simulink model "Robot_Protected_Model"  (Simulink 8.0)
settings: Solver=ode45  StartTime=0.0  StopTime=simtime  MaxStep=0.01  RelTol=1e-3
values from neighbouring files (symbols this model uses):
  de = 30*pi/180    (= 0.523598775598)    [Robot_Feedback_Master.m]
  de0 = 0    [Robot_Feedback_Master.m]
  F = [mu1, 0; 0, mu2]    [Robot_Feedback_Master.m]
  g = 9.81    [Robot_Feedback_Master.m]
  Gamma0 = 1*diag([1, 1, 1, 1, 1, 1, 1, 1, 1], 0)    [Robot_Feedback_Master.m]
  Gamma1 = 0.0*diag([1, 1, 1, 1, 1, 1, 1, 1, 1], 0)    [Robot_Feedback_Master.m]
  I1 = 0.12    [Robot_Feedback_Master.m]
  Ie = 0.25    [Robot_Feedback_Master.m]
  Ie0 = 0.12    [Robot_Feedback_Master.m]
  initial_pos = 1*[-3; -3]    [Robot_Feedback_Master.m]
  initial_theta = 0*theta'    [Robot_Feedback_Master.m]
  initial_vel = 1*[-6; 6]    [Robot_Feedback_Master.m]
  KD = 100 * eye(2, 2)    [Robot_Feedback_Master.m]
  L1 = 1    [Robot_Feedback_Master.m]
  lambda = 0    [Robot_Feedback_Master.m]
  Lambda = 10 * eye(2, 2)    [Robot_Feedback_Master.m]
  Lc1 = 0.5    [Robot_Feedback_Master.m]
  Lce = 0.6    [Robot_Feedback_Master.m]
  Lce0 = 0.5    [Robot_Feedback_Master.m]
  M1 = 1    [Robot_Feedback_Master.m]
  Me = 5    [Robot_Feedback_Master.m]
  Me0 = 1    [Robot_Feedback_Master.m]
  mu1 = 0*0.1    (= 0)    [Robot_Feedback_Master.m]
  mu10 = 0*0.2    (= 0)    [Robot_Feedback_Master.m]
  mu2 = 0*0.1    (= 0)    [Robot_Feedback_Master.m]
  mu20 = 0*0.2    (= 0)    [Robot_Feedback_Master.m]
  tau1lim = 500    [Robot_Feedback_Master.m]
  tau2lim = 250    [Robot_Feedback_Master.m]
  thetaeps = 10    [Robot_Feedback_Master.m]
  thetamax = 40    [Robot_Feedback_Master.m]
settings Model: Creator=Travis  LastModifiedBy=Dan
settings DataIOCC: SignalLoggingSaveFormat=ModelDataLogs
settings DebuggingCC: FcnCallInpInsideContextMsg=UseLocalSettings
settings GRTTargetCC: CombineOutputUpdateFcns=off  GRTInterface=on

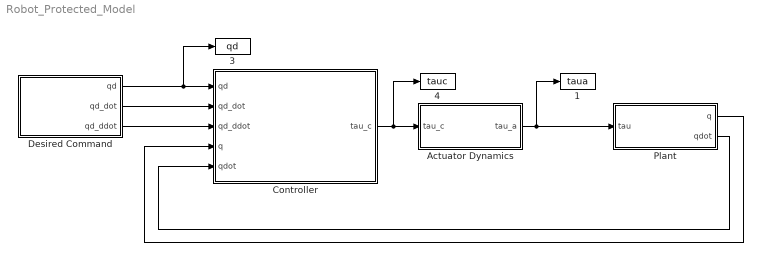
== system Robot_Protected_Model ==
  1 : ToWorkspace  VariableName=taua  SampleTime=-1  SaveFormat=Structure With Time
  3 : ToWorkspace  VariableName=qd  SampleTime=-1  SaveFormat=Structure With Time
  4 : ToWorkspace  VariableName=tauc  SampleTime=-1  SaveFormat=Structure With Time
  Actuator Dynamics : Subsystem
  Controller : Subsystem
  Desired Command : Subsystem
  Plant : Subsystem
  wires:
  Plant/2(qdot) -> Controller/5(qdot)
  Plant/1(q) -> Controller/4(q)
  Controller/1(tau_c) -> 4/1, Actuator Dynamics/1(tau_c)
  Desired Command/1(qd) -> 3/1, Controller/1(qd)
  Actuator Dynamics/1(tau_a) -> Plant/1(tau), 1/1
  Desired Command/2(qd_dot) -> Controller/2(qd_dot)
  Desired Command/3(qd_ddot) -> Controller/3(qd_ddot)

== system Robot_Protected_Model/Actuator Dynamics ==
  tau_c : Inport
  Demux : Demux  Outputs=2
  Mux : Mux  Inputs=2
  Saturation : Saturate  UpperLimit=tau1lim  LowerLimit=-tau1lim  ZeroCross=off
  Saturation1 : Saturate  UpperLimit=tau2lim  LowerLimit=-tau2lim  ZeroCross=off
  tau_a : Outport
  wires:
  Demux/1 -> Saturation/1
  Saturation/1 -> Mux/1
  Demux/2 -> Saturation1/1
  Saturation1/1 -> Mux/2
  Mux/1 -> tau_a/1
  tau_c/1 -> Demux/1

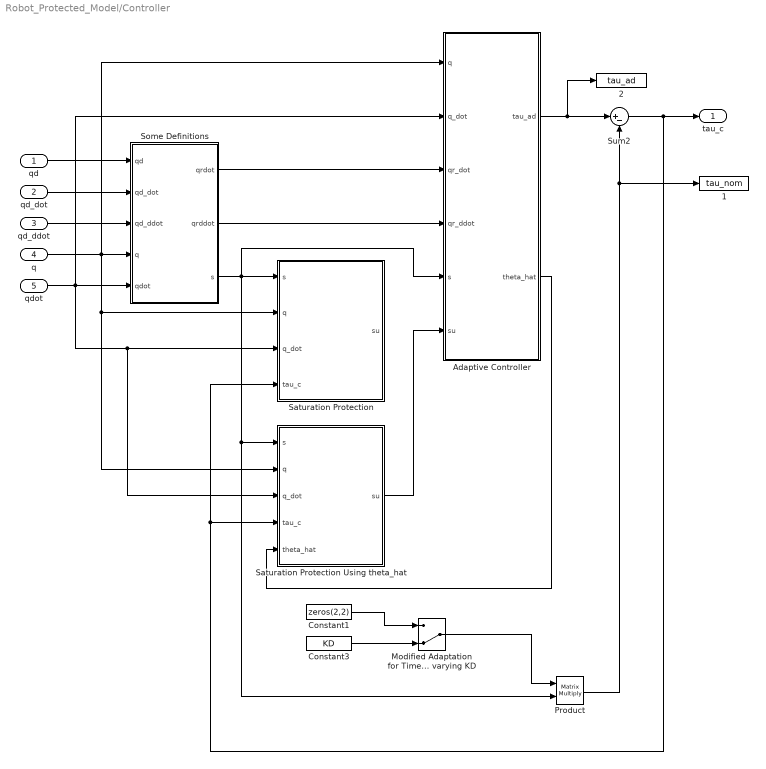
== system Robot_Protected_Model/Controller ==
  qd : Inport
  qd_dot : Inport  Port=2
  qd_ddot : Inport  Port=3
  q : Inport  Port=4
  qdot : Inport  Port=5
  1 : ToWorkspace  VariableName=tau_nom  SampleTime=-1  SaveFormat=Structure With Time
  2 : ToWorkspace  VariableName=tau_ad  SampleTime=-1  SaveFormat=Structure With Time
  Adaptive Controller : Subsystem
  Constant1 : Constant  Value=zeros(2,2)
  Constant3 : Constant  Value=KD
  Modified Adaptation for Time Varying KD (SWITCH 2 of 2) up is time varying KD : ManualSwitch  CurrentSetting=0
  Product : Product  Multiplication=Matrix(*)  RndMeth=Zero
  Saturation Protection : Subsystem
  Saturation Protection Using theta_hat : Subsystem
  Some Definitions : Subsystem
  Sum2 : Sum  Inputs=|+-
  tau_c : Outport
  wires:
  Adaptive Controller/1(tau_ad) -> 2/1, Sum2/1
  Product/1 -> 1/1, Sum2/2
  Sum2/1 -> tau_c/1, Saturation Protection/4(tau_c), Saturation Protection Using theta_hat/4(tau_c)
  q/1 -> Saturation Protection Using theta_hat/2(q), Saturation Protection/2(q), Some Definitions/4(q), Adaptive Controller/1(q)
  qdot/1 -> Adaptive Controller/2(q_dot), Saturation Protection Using theta_hat/3(q_dot), Saturation Protection/3(q_dot), Some Definitions/5(qdot)
  Some Definitions/1(qrdot) -> Adaptive Controller/3(qr_dot)
  Some Definitions/2(qrddot) -> Adaptive Controller/4(qr_ddot)
  qd_ddot/1 -> Some Definitions/3(qd_ddot)
  qd_dot/1 -> Some Definitions/2(qd_dot)
  qd/1 -> Some Definitions/1(qd)
  Some Definitions/3(s) -> Saturation Protection Using theta_hat/1(s), Product/2, Adaptive Controller/5(s), Saturation Protection/1(s)
  Constant3/1 -> Modified Adaptation for Time Varying KD (SWITCH 2 of 2) up is time varying KD/2
  Constant1/1 -> Modified Adaptation for Time Varying KD (SWITCH 2 of 2) up is time varying KD/1
  Modified Adaptation for Time Varying KD (SWITCH 2 of 2) up is time varying KD/1 -> Product/1
  Adaptive Controller/2(theta_hat) -> Saturation Protection Using theta_hat/5(theta_hat)
  Saturation Protection Using theta_hat/1(su) -> Adaptive Controller/6(su)

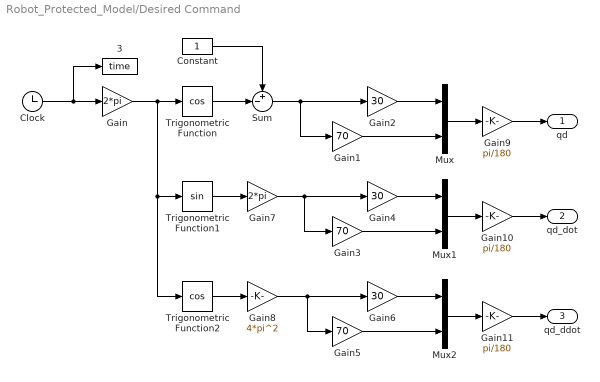
== system Robot_Protected_Model/Desired Command ==
  3 : ToWorkspace  VariableName=time  SampleTime=-1
  Clock : Clock
  Constant : Constant
  Gain : Gain  Gain=2*pi
  Gain1 : Gain  Gain=70
  Gain10 : Gain  Gain=pi/180
  Gain11 : Gain  Gain=pi/180
  Gain2 : Gain  Gain=30
  Gain3 : Gain  Gain=70
  Gain4 : Gain  Gain=30
  Gain5 : Gain  Gain=70
  Gain6 : Gain  Gain=30
  Gain7 : Gain  Gain=2*pi
  Gain8 : Gain  Gain=4*pi^2
  Gain9 : Gain  Gain=pi/180
  Mux : Mux  Inputs=2
  Mux1 : Mux  Inputs=2
  Mux2 : Mux  Inputs=2
  Sum : Sum  Inputs=+-|
  Trigonometric Function : Trigonometry  Operator=cos
  Trigonometric Function1 : Trigonometry
  Trigonometric Function2 : Trigonometry  Operator=cos
  qd : Outport
  qd_dot : Outport  Port=2
  qd_ddot : Outport  Port=3
  wires:
  Clock/1 -> Gain/1, 3/1
  Gain/1 -> Trigonometric Function/1, Trigonometric Function1/1, Trigonometric Function2/1
  Sum/1 -> Gain2/1, Gain1/1
  Gain1/1 -> Mux/2
  Trigonometric Function1/1 -> Gain7/1
  Trigonometric Function2/1 -> Gain8/1
  Mux/1 -> Gain9/1
  Gain2/1 -> Mux/1
  Gain7/1 -> Gain4/1, Gain3/1
  Gain3/1 -> Mux1/2
  Gain4/1 -> Mux1/1
  Gain8/1 -> Gain5/1, Gain6/1
  Gain5/1 -> Mux2/2
  Mux2/1 -> Gain11/1
  Gain6/1 -> Mux2/1
  Mux1/1 -> Gain10/1
  Constant/1 -> Sum/1
  Trigonometric Function/1 -> Sum/2
  Gain9/1 -> qd/1
  Gain10/1 -> qd_dot/1
  Gain11/1 -> qd_ddot/1

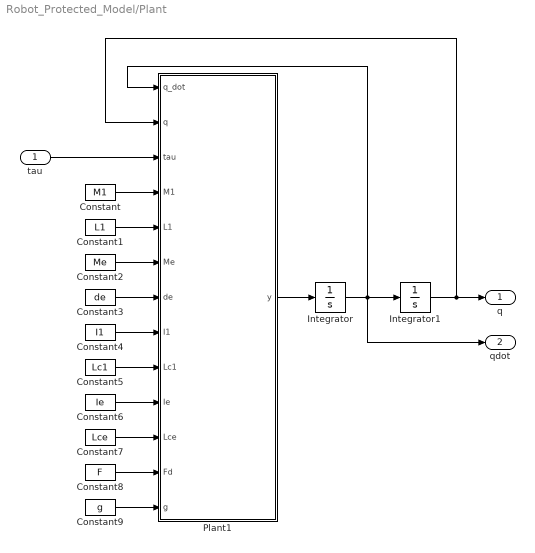
== system Robot_Protected_Model/Plant ==
  tau : Inport
  Constant : Constant  Value=M1
  Constant1 : Constant  Value=L1
  Constant2 : Constant  Value=Me
  Constant3 : Constant  Value=de
  Constant4 : Constant  Value=I1
  Constant5 : Constant  Value=Lc1
  Constant6 : Constant  Value=Ie
  Constant7 : Constant  Value=Lce
  Constant8 : Constant  Value=F
  Constant9 : Constant  Value=g
  Integrator : Integrator  InitialCondition=initial_vel
  Integrator1 : Integrator  InitialCondition=initial_pos
  Plant1 : MATLAB Function  TreatAsAtomicUnit=on
  q : Outport
  qdot : Outport  Port=2
  wires:
  Plant1/1(y) -> Integrator/1
  Integrator/1 -> qdot/1, Plant1/1(q_dot), Integrator1/1
  Constant/1 -> Plant1/4(M1)
  Constant1/1 -> Plant1/5(L1)
  Constant2/1 -> Plant1/6(Me)
  Constant3/1 -> Plant1/7(de)
  Constant5/1 -> Plant1/9(Lc1)
  Constant4/1 -> Plant1/8(I1)
  Constant6/1 -> Plant1/10(Ie)
  Constant7/1 -> Plant1/11(Lce)
  tau/1 -> Plant1/3(tau)
  Integrator1/1 -> Plant1/2(q), q/1
  Constant8/1 -> Plant1/12(Fd)
  Constant9/1 -> Plant1/13(g)

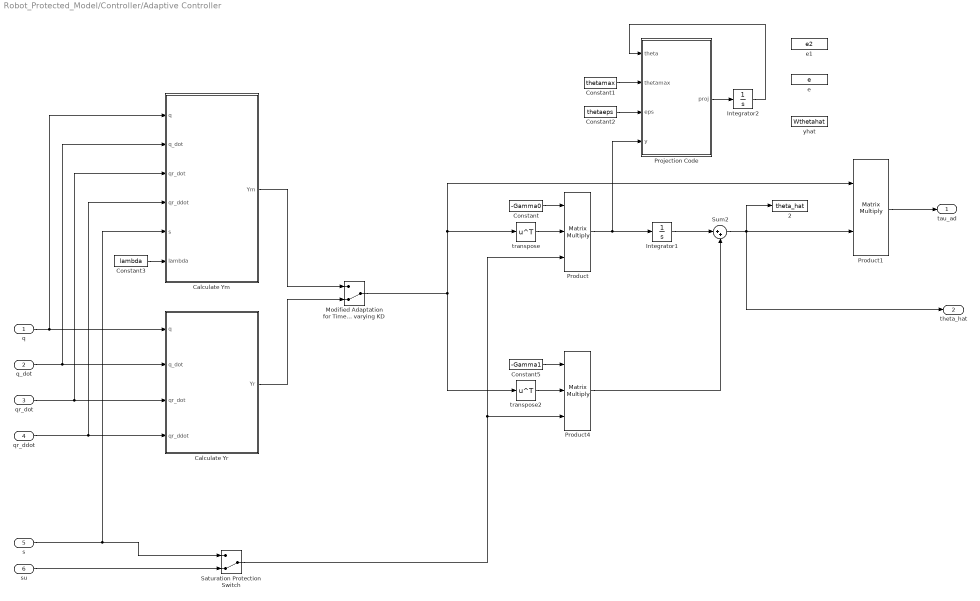
== system Robot_Protected_Model/Controller/Adaptive Controller ==
  q : Inport
  q_dot : Inport  Port=2
  qr_dot : Inport  Port=3
  qr_ddot : Inport  Port=4
  s : Inport  Port=5
  su : Inport  Port=6
  2 : ToWorkspace  VariableName=theta_hat  SampleTime=-1  SaveFormat=Structure With Time
  Calculate Ym : MATLAB Function  TreatAsAtomicUnit=on
  Calculate Yr : MATLAB Function  TreatAsAtomicUnit=on
  Constant : Constant  Value=-Gamma0
  Constant1 : Constant  Value=thetamax
  Constant2 : Constant  Value=thetaeps
  Constant3 : Constant  Value=lambda
  Constant5 : Constant  Value=-Gamma1
  Integrator1 : Integrator  InitialCondition=initial_theta
  Integrator2 : Integrator  InitialCondition=initial_theta
  Modified Adaptation for Time Varying KD (SWITCH 1 of 2) up is time varying KD : ManualSwitch  CurrentSetting=0
  Product : Product  Inputs=3  Multiplication=Matrix(*)  RndMeth=Zero
  Product1 : Product  Multiplication=Matrix(*)  RndMeth=Zero
  Product4 : Product  Inputs=3  Multiplication=Matrix(*)  RndMeth=Zero
  Projection Code : Subsystem
  Saturation Protection Switch : ManualSwitch  CurrentSetting=0
  Sum2 : Sum  Inputs=|++
  e : ToWorkspace  VariableName=e  SampleTime=-1  SaveFormat=Structure With Time
  e1 : ToWorkspace  VariableName=e2  SampleTime=-1  SaveFormat=Structure With Time
  transpose : Math  Operator=transpose  SaturateOnIntegerOverflow=on
  transpose2 : Math  Operator=transpose  SaturateOnIntegerOverflow=on
  yhat : ToWorkspace  VariableName=Wthetahat  SampleTime=-1  SaveFormat=Structure With Time
  tau_ad : Outport
  theta_hat : Outport  Port=2
  wires:
  Constant/1 -> Product/1
  transpose/1 -> Product/2
  Product1/1 -> tau_ad/1
  q/1 -> Calculate Yr/1(q), Calculate Ym/1(q)
  qr_ddot/1 -> Calculate Ym/4(qr_ddot), Calculate Yr/4(qr_ddot)
  qr_dot/1 -> Calculate Ym/3(qr_dot), Calculate Yr/3(qr_dot)
  q_dot/1 -> Calculate Ym/2(q_dot), Calculate Yr/2(q_dot)
  s/1 -> Calculate Ym/5(s), Saturation Protection Switch/1
  su/1 -> Saturation Protection Switch/2
  Saturation Protection Switch/1 -> Product4/3, Product/3
  Constant3/1 -> Calculate Ym/6(lambda)
  Modified Adaptation for Time Varying KD (SWITCH 1 of 2) up is time varying KD/1 -> transpose/1, Product1/1, transpose2/1
  Calculate Ym/1(Ym) -> Modified Adaptation for Time Varying KD (SWITCH 1 of 2) up is time varying KD/1
  Calculate Yr/1(Yr) -> Modified Adaptation for Time Varying KD (SWITCH 1 of 2) up is time varying KD/2
  Projection Code/1(proj) -> Integrator2/1
  Constant1/1 -> Projection Code/2(thetamax)
  Constant2/1 -> Projection Code/3(eps)
  Sum2/1 -> theta_hat/1, Product1/2, 2/1
  Product/1 -> Projection Code/4(y), Integrator1/1
  Integrator2/1 -> Projection Code/1(theta)
  Constant5/1 -> Product4/1
  transpose2/1 -> Product4/2
  Product4/1 -> Sum2/2
  Integrator1/1 -> Sum2/1

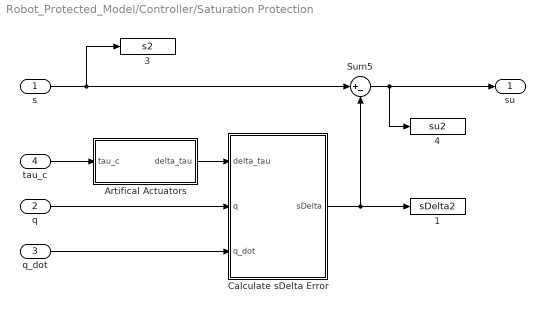
== system Robot_Protected_Model/Controller/Saturation Protection ==
  s : Inport
  q : Inport  Port=2
  q_dot : Inport  Port=3
  tau_c : Inport  Port=4
  1 : ToWorkspace  VariableName=sDelta2  SampleTime=-1  SaveFormat=Structure With Time
  3 : ToWorkspace  VariableName=s2  SampleTime=-1  SaveFormat=Structure With Time
  4 : ToWorkspace  VariableName=su2  SampleTime=-1  SaveFormat=Structure With Time
  Artifical Actuators : Subsystem
  "Calculate sDelta Error " : Subsystem
  Sum5 : Sum  Inputs=|+-
  su : Outport
  wires:
  q/1 -> "Calculate sDelta Error "/2(q)
  q_dot/1 -> "Calculate sDelta Error "/3(q_dot)
  Artifical Actuators/1(delta_tau) -> "Calculate sDelta Error "/1(delta_tau)
  s/1 -> 3/1, Sum5/1
  Sum5/1 -> su/1, 4/1
  "Calculate sDelta Error "/1(sDelta) -> 1/1, Sum5/2
  tau_c/1 -> Artifical Actuators/1(tau_c)

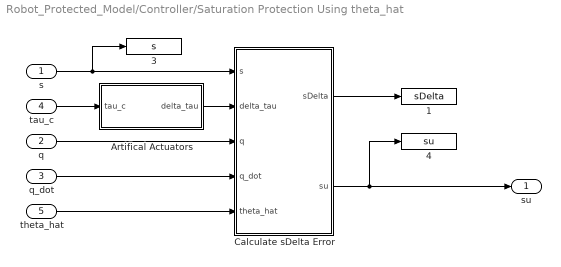
== system Robot_Protected_Model/Controller/Saturation Protection Using theta_hat ==
  s : Inport
  q : Inport  Port=2
  q_dot : Inport  Port=3
  tau_c : Inport  Port=4
  theta_hat : Inport  Port=5
  1 : ToWorkspace  VariableName=sDelta  SampleTime=-1  SaveFormat=Structure With Time
  3 : ToWorkspace  VariableName=s  SampleTime=-1  SaveFormat=Structure With Time
  4 : ToWorkspace  VariableName=su  SampleTime=-1  SaveFormat=Structure With Time
  Artifical Actuators : Subsystem
  "Calculate sDelta Error " : Subsystem
  su : Outport
  wires:
  q/1 -> "Calculate sDelta Error "/3(q)
  q_dot/1 -> "Calculate sDelta Error "/4(q_dot)
  Artifical Actuators/1(delta_tau) -> "Calculate sDelta Error "/2(delta_tau)
  s/1 -> 3/1, "Calculate sDelta Error "/1(s)
  "Calculate sDelta Error "/1(sDelta) -> 1/1
  tau_c/1 -> Artifical Actuators/1(tau_c)
  theta_hat/1 -> "Calculate sDelta Error "/5(theta_hat)
  "Calculate sDelta Error "/2(su) -> su/1, 4/1

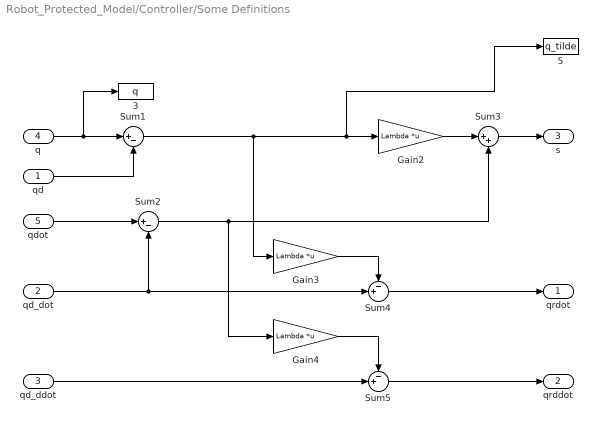
== system Robot_Protected_Model/Controller/Some Definitions ==
  qd : Inport
  qd_dot : Inport  Port=2
  qd_ddot : Inport  Port=3
  q : Inport  Port=4
  qdot : Inport  Port=5
  3 : ToWorkspace  VariableName=q  SampleTime=-1  SaveFormat=Structure With Time
  5 : ToWorkspace  VariableName=q_tilde  SampleTime=-1  SaveFormat=Structure With Time
  Gain2 : Gain  Gain=Lambda  Multiplication=Matrix(K*u)
  Gain3 : Gain  Gain=Lambda  Multiplication=Matrix(K*u)
  Gain4 : Gain  Gain=Lambda  Multiplication=Matrix(K*u)
  Sum1 : Sum  Inputs=|+-
  Sum2 : Sum  Inputs=|+-
  Sum3 : Sum  Inputs=|++
  Sum4 : Sum  Inputs=-+|
  Sum5 : Sum  Inputs=-+|
  qrdot : Outport
  qrddot : Outport  Port=2
  s : Outport  Port=3
  wires:
  qd/1 -> Sum1/2
  qd_dot/1 -> Sum2/2, Sum4/2
  q/1 -> 3/1, Sum1/1
  Sum1/1 -> Gain3/1, 5/1, Gain2/1
  qdot/1 -> Sum2/1
  Sum2/1 -> Sum3/2, Gain4/1
  Gain2/1 -> Sum3/1
  Sum3/1 -> s/1
  Sum4/1 -> qrdot/1
  Sum5/1 -> qrddot/1
  Gain3/1 -> Sum4/1
  Gain4/1 -> Sum5/1
  qd_ddot/1 -> Sum5/2

== system Robot_Protected_Model/Controller/Adaptive Controller/Projection Code ==
  note: This block is the projection operator. See notes.
  theta : Inport
  thetamax : Inport  Port=2
  eps : Inport  Port=3
  y : Inport  Port=4
  Projection : MATLAB Function  TreatAsAtomicUnit=on
  proj : Outport
  wires:
  Projection/1(proj) -> proj/1
  theta/1 -> Projection/1(theta)
  thetamax/1 -> Projection/2(thetamax)
  eps/1 -> Projection/3(eps)
  y/1 -> Projection/4(y)

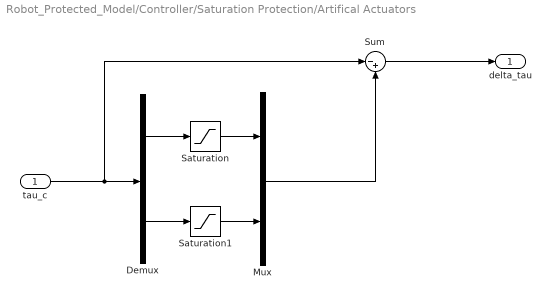
== system Robot_Protected_Model/Controller/Saturation Protection/Artifical Actuators ==
  tau_c : Inport
  Demux : Demux  Outputs=2
  Mux : Mux  Inputs=2
  Saturation : Saturate  UpperLimit=tau1lim  LowerLimit=-tau1lim  ZeroCross=off
  Saturation1 : Saturate  UpperLimit=tau2lim  LowerLimit=-tau2lim  ZeroCross=off
  Sum : Sum  Inputs=|-+
  delta_tau : Outport
  wires:
  Demux/1 -> Saturation/1
  Saturation/1 -> Mux/1
  Demux/2 -> Saturation1/1
  Saturation1/1 -> Mux/2
  tau_c/1 -> Sum/1, Demux/1
  Mux/1 -> Sum/2
  Sum/1 -> delta_tau/1

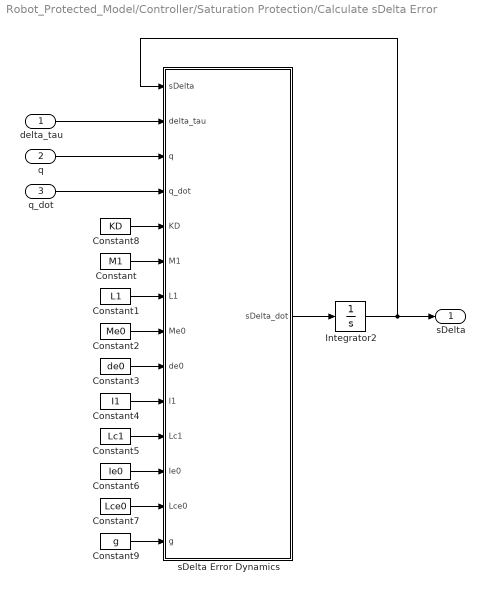
== system Robot_Protected_Model/Controller/Saturation Protection/Calculate sDelta Error  ==
  delta_tau : Inport
  q : Inport  Port=2
  q_dot : Inport  Port=3
  Constant : Constant  Value=M1
  Constant1 : Constant  Value=L1
  Constant2 : Constant  Value=Me0
  Constant3 : Constant  Value=de0
  Constant4 : Constant  Value=I1
  Constant5 : Constant  Value=Lc1
  Constant6 : Constant  Value=Ie0
  Constant7 : Constant  Value=Lce0
  Constant8 : Constant  Value=KD
  Constant9 : Constant  Value=g
  Integrator2 : Integrator  InitialCondition=[0;0];
  sDelta Error Dynamics : MATLAB Function  TreatAsAtomicUnit=on
  sDelta : Outport
  wires:
  delta_tau/1 -> sDelta Error Dynamics/2(delta_tau)
  sDelta Error Dynamics/1(sDelta_dot) -> Integrator2/1
  Integrator2/1 -> sDelta Error Dynamics/1(sDelta), sDelta/1
  Constant/1 -> sDelta Error Dynamics/6(M1)
  Constant1/1 -> sDelta Error Dynamics/7(L1)
  Constant2/1 -> sDelta Error Dynamics/8(Me0)
  Constant3/1 -> sDelta Error Dynamics/9(de0)
  Constant4/1 -> sDelta Error Dynamics/10(I1)
  Constant5/1 -> sDelta Error Dynamics/11(Lc1)
  Constant6/1 -> sDelta Error Dynamics/12(Ie0)
  Constant7/1 -> sDelta Error Dynamics/13(Lce0)
  q/1 -> sDelta Error Dynamics/3(q)
  q_dot/1 -> sDelta Error Dynamics/4(q_dot)
  Constant8/1 -> sDelta Error Dynamics/5(KD)
  Constant9/1 -> sDelta Error Dynamics/14(g)

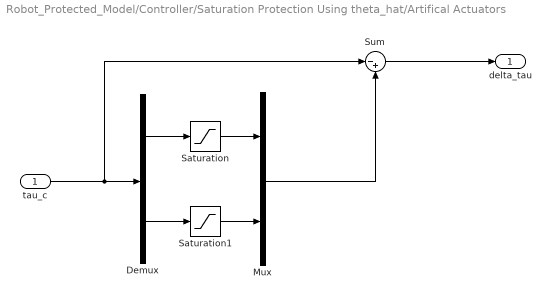
== system Robot_Protected_Model/Controller/Saturation Protection Using theta_hat/Artifical Actuators ==
  tau_c : Inport
  Demux : Demux  Outputs=2
  Mux : Mux  Inputs=2
  Saturation : Saturate  UpperLimit=tau1lim  LowerLimit=-tau1lim  ZeroCross=off
  Saturation1 : Saturate  UpperLimit=tau2lim  LowerLimit=-tau2lim  ZeroCross=off
  Sum : Sum  Inputs=|-+
  delta_tau : Outport
  wires:
  Demux/1 -> Saturation/1
  Saturation/1 -> Mux/1
  Demux/2 -> Saturation1/1
  Saturation1/1 -> Mux/2
  tau_c/1 -> Sum/1, Demux/1
  Mux/1 -> Sum/2
  Sum/1 -> delta_tau/1

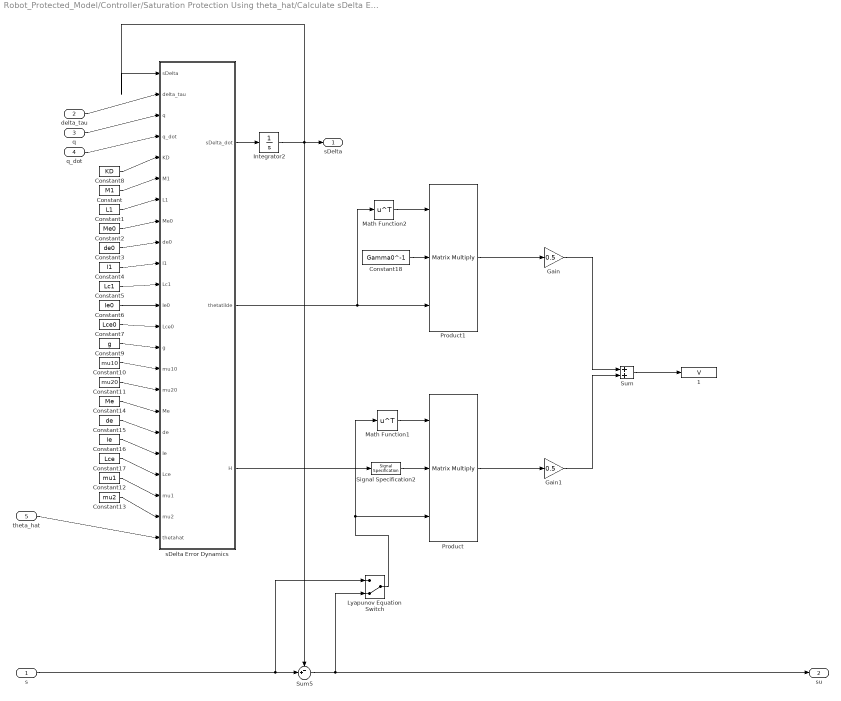
== system Robot_Protected_Model/Controller/Saturation Protection Using theta_hat/Calculate sDelta Error  ==
  s : Inport
  delta_tau : Inport  Port=2
  q : Inport  Port=3
  q_dot : Inport  Port=4
  theta_hat : Inport  Port=5
  1 : ToWorkspace  VariableName=V  SampleTime=-1  SaveFormat=Structure With Time
  Constant : Constant  Value=M1
  Constant1 : Constant  Value=L1
  Constant10 : Constant  Value=mu10
  Constant11 : Constant  Value=mu20
  Constant12 : Constant  Value=mu1
  Constant13 : Constant  Value=mu2
  Constant14 : Constant  Value=Me
  Constant15 : Constant  Value=de
  Constant16 : Constant  Value=Ie
  Constant17 : Constant  Value=Lce
  Constant18 : Constant  Value=Gamma0^-1
  Constant2 : Constant  Value=Me0
  Constant3 : Constant  Value=de0
  Constant4 : Constant  Value=I1
  Constant5 : Constant  Value=Lc1
  Constant6 : Constant  Value=Ie0
  Constant7 : Constant  Value=Lce0
  Constant8 : Constant  Value=KD
  Constant9 : Constant  Value=g
  Gain : Gain  Gain=0.5
  Gain1 : Gain  Gain=0.5
  Integrator2 : Integrator  InitialCondition=[0;0];
  Lyapunov Equation Switch : ManualSwitch  CurrentSetting=0
  Math Function1 : Math  Operator=transpose  SaturateOnIntegerOverflow=on
  Math Function2 : Math  Operator=transpose  SaturateOnIntegerOverflow=on
  Product : Product  Inputs=3  Multiplication=Matrix(*)  RndMeth=Zero
  Product1 : Product  Inputs=3  Multiplication=Matrix(*)  RndMeth=Zero
  Signal Specification2 : SignalSpecification  Dimensions=[2 2]
  Sum : Sum
  Sum5 : Sum  Inputs=-+|
  sDelta Error Dynamics : MATLAB Function  TreatAsAtomicUnit=on
  sDelta : Outport
  su : Outport  Port=2
  wires:
  delta_tau/1 -> sDelta Error Dynamics/2(delta_tau)
  sDelta Error Dynamics/1(sDelta_dot) -> Integrator2/1
  Integrator2/1 -> sDelta Error Dynamics/1(sDelta), Sum5/1, sDelta/1
  Constant/1 -> sDelta Error Dynamics/6(M1)
  Constant1/1 -> sDelta Error Dynamics/7(L1)
  Constant2/1 -> sDelta Error Dynamics/8(Me0)
  Constant3/1 -> sDelta Error Dynamics/9(de0)
  Constant4/1 -> sDelta Error Dynamics/10(I1)
  Constant5/1 -> sDelta Error Dynamics/11(Lc1)
  Constant6/1 -> sDelta Error Dynamics/12(Ie0)
  Constant7/1 -> sDelta Error Dynamics/13(Lce0)
  q/1 -> sDelta Error Dynamics/3(q)
  q_dot/1 -> sDelta Error Dynamics/4(q_dot)
  Constant8/1 -> sDelta Error Dynamics/5(KD)
  Constant9/1 -> sDelta Error Dynamics/14(g)
  theta_hat/1 -> sDelta Error Dynamics/23(thetahat)
  s/1 -> Lyapunov Equation Switch/1, Sum5/2
  Constant10/1 -> sDelta Error Dynamics/15(mu10)
  Constant11/1 -> sDelta Error Dynamics/16(mu20)
  Constant14/1 -> sDelta Error Dynamics/17(Me)
  Constant15/1 -> sDelta Error Dynamics/18(de)
  Constant16/1 -> sDelta Error Dynamics/19(Ie)
  Constant17/1 -> sDelta Error Dynamics/20(Lce)
  Constant12/1 -> sDelta Error Dynamics/21(mu1)
  Constant13/1 -> sDelta Error Dynamics/22(mu2)
  Sum5/1 -> Lyapunov Equation Switch/2, su/1
  sDelta Error Dynamics/3(H) -> Signal Specification2/1
  Signal Specification2/1 -> Product/2
  Math Function1/1 -> Product/1
  Constant18/1 -> Product1/2
  sDelta Error Dynamics/2(thetatilde) -> Product1/3, Math Function2/1
  Math Function2/1 -> Product1/1
  Product/1 -> Gain1/1
  Product1/1 -> Gain/1
  Sum/1 -> 1/1
  Gain/1 -> Sum/1
  Gain1/1 -> Sum/2
  Lyapunov Equation Switch/1 -> Product/3, Math Function1/1

== matlab function Controller/Adaptive Controller/Calculate Yr ==
  data: q input double; q_dot input double; qr_dot input double; qr_ddot input double; Yr output double
%%%%%%%%%%%%%%%%%%%%%%%%%%%%%%%%%%%%%%%%%%%%%%%%%%%%%%%%%%%%%%%%%%%%%%%%%%%
% Daniel Wiese
% 2.152
% Robot Manipulator
%--------------------------------------------------------------------------
% Robot
%%%%%%%%%%%%%%%%%%%%%%%%%%%%%%%%%%%%%%%%%%%%%%%%%%%%%%%%%%%%%%%%%%%%%%%%%%%
function Yr=fcn(q,q_dot,qr_dot,qr_ddot)
%#codegen
%Preallocate output
Yr=zeros(2,9);
%Take apart the input
q1=q(1);
q2=q(2);
q_dot1=q_dot(1);
q_dot2=q_dot(2);
qr_dot1=qr_dot(1);
qr_dot2=qr_dot(2);
qr_ddot1=qr_ddot(1);
qr_ddot2=qr_ddot(2);
%Calculate the first row of Y
Yr(1,1)=qr_ddot1;
Yr(1,2)=qr_ddot2;
Yr(1,3)=(2*qr_ddot1+qr_ddot2)*cos(q2)-(q_dot2*qr_dot1+q_dot1*qr_dot2+q_dot2*qr_dot2)*sin(q2);
Yr(1,4)=(2*qr_ddot1+qr_ddot2)*sin(q2)+(q_dot2*qr_dot1+q_dot1*qr_dot2+q_dot2*qr_dot2)*cos(q2);
Yr(1,5)=cos(q1);
Yr(1,6)=cos(q1+q2);
Yr(1,7)=-sin(q1+q2);
Yr(1,8)=q_dot1;
Yr(1,9)=0;
%Calculate the second row of Y
Yr(2,1)=0;
Yr(2,2)=qr_ddot1+qr_ddot2;
Yr(2,3)=qr_ddot1*cos(q2)+q_dot1*qr_dot1*sin(q2);
Yr(2,4)=qr_ddot1*sin(q2)-q_dot1*qr_dot1*cos(q2);
Yr(2,5)=0;
Yr(2,6)=cos(q1+q2);
Yr(2,7)=-sin(q1+q2);
Yr(2,8)=0;
Yr(2,9)=q_dot2;

== matlab function Controller/Saturation Protection/Calculate sDelta Error /sDelta Error Dynamics ==
  data: sDelta input double; sDelta_dot output double; delta_tau input double; q input double; q_dot input double; KD input double; M1 input double; L1 input double; Me0 input double; de0 input double; I1 input double; Lc1 input double; Ie0 input double; Lce0 input double; g input double
%%%%%%%%%%%%%%%%%%%%%%%%%%%%%%%%%%%%%%%%%%%%%%%%%%%%%%%%%%%%%%%%%%%%%%%%%%%
% Daniel Wiese
% 2.152
% Robot Manipulator
%--------------------------------------------------------------------------
% Robot manipulator. See Slotine, Li page 396 for the equations and all of
% the parameter values used.
%%%%%%%%%%%%%%%%%%%%%%%%%%%%%%%%%%%%%%%%%%%%%%%%%%%%%%%%%%%%%%%%%%%%%%%%%%%
function sDelta_dot = fcn(sDelta,delta_tau,q,q_dot,KD,M1,L1,Me0,de0,I1,Lc1,Ie0,Lce0,g)
%#codegen
%Take apart the input
q1=q(1);
q2=q(2);
qdot1=q_dot(1);
qdot2=q_dot(2);
%Define the nominal parameters
theta1=I1+M1*Lc1^2+Ie0+Me0*Lc1^2+Me0*L1^2;
theta2=Ie0+Me0*Lce0^2;
theta3=Me0*L1*Lce0*cos(de0);
theta4=Me0*L1*Lce0*sin(de0);
%Components of the matrix H
H11=theta1+2*theta3*cos(q2)+2*theta4*sin(q2);
H12=theta2+theta3*cos(q2)+theta4*sin(q2);
H21=H12;
H22=theta2;
h=theta3*sin(q2)-theta4*cos(q2);
%The gravity matrix G
G=[(M1*Lc1+Me0*L1)*g*cos(q1)+((Me0*Lce0*g)/cos(de0))*cos(q1+q2+de0);
    ((Me0*Lce0*g)/cos(de0))*cos(q1+q2+de0)];
%Assemble H and C
H=[H11 H12; H21 H22];
C=[-h*qdot2 -h*(qdot1+qdot2); h*qdot1 0];
%Calculate sDelta
sDelta_dot=-H\(C+KD)*sDelta+H\delta_tau;
% sDelta_dot=-10*eye(2,2)*sDelta+0.1*eye(2,2)*delta_tau;

== matlab function Controller/Adaptive Controller/Projection Code/Projection ==
  data: theta input double; thetamax input double; eps input double; proj output double; y input double
%%%%%%%%%%%%%%%%%%%%%%%%%%%%%%%%%%%%%%%%%%%%%%%%%%%%%%%%%%%%%%%%%%%%%%%%%%%
% Daniel Wiese
% Generic Hypersonic Vehicle
% Projection Operator
% 2012-06-05
%--------------------------------------------------------------------------
% This function is the projection algorithm for use in an adaptive control
% law. The inputs are the outer ball radius, and inner radius scaling 
% factor epsilon, which determines the inner radius of the ball. See notes
% for more information.
%%%%%%%%%%%%%%%%%%%%%%%%%%%%%%%%%%%%%%%%%%%%%%%%%%%%%%%%%%%%%%%%%%%%%%%%%%%
function proj=projection(theta,thetamax,eps,y)
%Preallocate
[n,m]=size(theta);
f=zeros(m,1);
gradf=zeros(n,m);
proj=zeros(n,m);
cond=zeros(m,1);
%Projection
for i=1:m
    f(i)=(norm(theta(:,i),2)^2-thetamax(i)^2)/(2*eps(i)*thetamax(i)+eps(i)^2);
    for j=1:n
        gradf(j,i)=(2*theta(j,i))/(2*eps(i)*thetamax(i)+eps(i)^2);
    end
    cond(i)=(f(i)>0 && y(:,i)'*gradf(:,i)>0 );
    if cond(i);
        proj(:,i)=y(:,i)-(gradf(:,i)*gradf(:,i)')/(gradf(:,i)'*gradf(:,i))*y(:,i)*f(i);
    else
        proj(:,i)=y(:,i);
    end
end
%%%%%%%%%%%%%%%%%%%%%%%%%%%%%%%%%%%%%%%%%%%%%%%%%%%%%%%%%%%%%%%%%%%%%%%%%%%

== matlab function Plant/Plant1 ==
  data: q_dot input double; q input double; y output double; tau input double; M1 input double; L1 input double; Me input double; de input double; I1 input double; Lc1 input double; Ie input double; Lce input double; Fd input double; g input double
%%%%%%%%%%%%%%%%%%%%%%%%%%%%%%%%%%%%%%%%%%%%%%%%%%%%%%%%%%%%%%%%%%%%%%%%%%%
% Daniel Wiese
% 2.152
% Robot Manipulator
%--------------------------------------------------------------------------
% Robot manipulator. See Slotine, Li page 396 for the equations and all of
% the parameter values used.
%%%%%%%%%%%%%%%%%%%%%%%%%%%%%%%%%%%%%%%%%%%%%%%%%%%%%%%%%%%%%%%%%%%%%%%%%%%
function y = fcn(q_dot,q,tau,M1,L1,Me,de,I1,Lc1,Ie,Lce,Fd,g)
%#codegen
%Take apart the input
q1=q(1);
q2=q(2);
qdot1=q_dot(1);
qdot2=q_dot(2);
%Define the 'a' parameters
a1=I1+M1*Lc1^2+Ie+Me*Lc1^2+Me*L1^2;
a2=Ie+Me*Lce^2;
a3=Me*L1*Lce*cos(de);
a4=Me*L1*Lce*sin(de);
%Components of the matrix H
H11=a1+2*a3*cos(q2)+2*a4*sin(q2);
H12=a2+a3*cos(q2)+a4*sin(q2);
H21=H12;
H22=a2;
h=a3*sin(q2)-a4*cos(q2);
%The gravity matrix G
G=[(M1*Lc1+Me*L1)*g*cos(q1)+((Me*Lce*g)/cos(de))*cos(q1+q2+de);
    ((Me*Lce*g)/cos(de))*cos(q1+q2+de)];
%Assemble H and C
H=[H11 H12; H21 H22];
C=[-h*qdot2 -h*(qdot1+qdot2); h*qdot1 0];
%Calculate the plant output y=q_ddot
y = -(H\C)*q_dot-(H\G)-(H\Fd)*q_dot+inv(H)*tau;

== matlab function Controller/Adaptive Controller/Calculate Ym ==
  data: q input double; q_dot input double; qr_dot input double; qr_ddot input double; s input double; lambda input double; Ym output double
%%%%%%%%%%%%%%%%%%%%%%%%%%%%%%%%%%%%%%%%%%%%%%%%%%%%%%%%%%%%%%%%%%%%%%%%%%%
% Daniel Wiese
% 2.152
% Robot Manipulator
%--------------------------------------------------------------------------
% Robot
%%%%%%%%%%%%%%%%%%%%%%%%%%%%%%%%%%%%%%%%%%%%%%%%%%%%%%%%%%%%%%%%%%%%%%%%%%%
function Ym=fcn(q,q_dot,qr_dot,qr_ddot,s,lambda)
%#codegen
%Preallocate output
Ym=zeros(2,9);
%Take apart the input
q1=q(1);
q2=q(2);
q_dot1=q_dot(1);
q_dot2=q_dot(2);
qr_dot1=qr_dot(1);
qr_dot2=qr_dot(2);
qr_ddot1=qr_ddot(1);
qr_ddot2=qr_ddot(2);
Ls1=lambda*s(1);
Ls2=lambda*s(2);
qr_ddot1=qr_ddot(1)-Ls1;
qr_ddot2=qr_ddot(2)-Ls2;
%Calculate the first row of Y
Ym(1,1)=qr_ddot1;
Ym(1,2)=qr_ddot2;
Ym(1,3)=(2*qr_ddot1+qr_ddot2)*cos(q2)-(q_dot2*qr_dot1+q_dot1*qr_dot2+q_dot2*qr_dot2)*sin(q2);
Ym(1,4)=(2*qr_ddot1+qr_ddot2)*sin(q2)+(q_dot2*qr_dot1+q_dot1*qr_dot2+q_dot2*qr_dot2)*cos(q2);
Ym(1,5)=cos(q1);
Ym(1,6)=cos(q1+q2);
Ym(1,7)=-sin(q1+q2);
Ym(1,8)=q_dot1;
Ym(1,9)=0;
%Calculate the second row of Y
Ym(2,1)=0;
Ym(2,2)=qr_ddot1+qr_ddot2;
Ym(2,3)=qr_ddot1*cos(q2)+q_dot1*qr_dot1*sin(q2);
Ym(2,4)=qr_ddot1*sin(q2)-q_dot1*qr_dot1*cos(q2);
Ym(2,5)=0;
Ym(2,6)=cos(q1+q2);
Ym(2,7)=-sin(q1+q2);
Ym(2,8)=0;
Ym(2,9)=q_dot2;

== matlab function Controller/Saturation Protection Using theta_hat/Calculate sDelta Error /sDelta Error Dynamics ==
  data: sDelta input double; sDelta_dot output double; delta_tau input double; q input double; q_dot input double; KD input double; M1 input double; L1 input double; Me0 input double; de0 input double; I1 input double; Lc1 input double; Ie0 input double; Lce0 input double; g input double; mu10 input double; mu20 input double; Me input double; de input double; Ie input double; Lce input double; mu1 input double; mu2 input double; thetahat input double; thetatilde output double; H output double
%%%%%%%%%%%%%%%%%%%%%%%%%%%%%%%%%%%%%%%%%%%%%%%%%%%%%%%%%%%%%%%%%%%%%%%%%%%
% Daniel Wiese
% 2.152
% Robot Manipulator
%--------------------------------------------------------------------------
% Robot manipulator. See Slotine, Li page 396 for the equations and all of
% the parameter values used.
%%%%%%%%%%%%%%%%%%%%%%%%%%%%%%%%%%%%%%%%%%%%%%%%%%%%%%%%%%%%%%%%%%%%%%%%%%%
function [sDelta_dot,thetatilde,H]=fcn(sDelta,delta_tau,q,q_dot,KD,M1,L1,Me0,de0,I1,Lc1,Ie0,Lce0,g,mu10,mu20,Me,de,Ie,Lce,mu1,mu2,thetahat)
%#codegen
%Take apart the input
q1=q(1);
q2=q(2);
qdot1=q_dot(1);
qdot2=q_dot(2);
%Define nominal parameter values
theta10=I1+M1*Lc1^2+Ie0+Me0*Lce0^2+Me0*L1^2; 
theta20=Ie0+Me0*Lce0^2; 
theta30=Me0*L1*Lce0*cos(de0); 
theta40=Me0*L1*Lce0*sin(de0);
theta50=(M1*Lc1+Me0*L1)*g;
theta60=Me0*Lce0*g;
theta70=Me0*Lce0*g*tan(de0);
theta80=mu10;
theta90=mu20;
%Actual parameter values
theta1=I1+M1*Lc1^2+Ie+Me*Lce^2+Me*L1^2; 
theta2=Ie+Me*Lce^2; 
theta3=Me*L1*Lce*cos(de); 
theta4=Me*L1*Lce*sin(de);
theta5=(M1*Lc1+Me*L1)*g;
theta6=Me*Lce*g;
theta7=Me*Lce*g*tan(de);
theta8=mu1;
theta9=mu2;
%Assemble these into vector
theta=[theta1 theta2 theta3 theta4 theta5 theta6 theta7 theta8 theta9];
theta0=[theta10 theta20 theta30 theta40 theta50 theta60 theta70 theta80 theta90];
thetatilde=thetahat-theta';

% %Use estimated parameters instead
% theta10=thetahat(1);
% theta20=thetahat(2);
% theta30=thetahat(3);
% theta40=thetahat(4);
% theta50=thetahat(5);
% theta60=thetahat(6);
% theta70=thetahat(7);
% theta80=thetahat(8);
% theta90=thetahat(9);

%Components of the matrix H nominal
H110=theta10+2*theta30*cos(q2)+2*theta40*sin(q2);
H120=theta20+theta30*cos(q2)+theta40*sin(q2);
H210=H120;
H220=theta20;
h0=theta30*sin(q2)-theta40*cos(q2);
%Components of the matrix H actual
H11=theta1+2*theta3*cos(q2)+2*theta4*sin(q2);
H12=theta2+theta3*cos(q2)+theta4*sin(q2);
H21=H12;
H22=theta2;
h=theta3*sin(q2)-theta4*cos(q2);




% %The gravity matrix G
% G=[(M1*Lc1+Me0*L1)*g*cos(q1)+((Me0*Lce0*g)/cos(de0))*cos(q1+q2+de0);
%     ((Me0*Lce0*g)/cos(de0))*cos(q1+q2+de0)];
%The gravity matrix G using estimated parameters
% G=[theta5*cos(q1)+theta6*cos(q1+q2)-theta7*sin(q1+q2);
%     theta6*cos(q1+q2)-theta7*sin(q1+q2)];

%Assemble H and C
H=[H11 H12; H21 H22];
H0=[H110 H120; H210 H220];
C=[-h*qdot2 -h*(qdot1+qdot2); h*qdot1 0];
C0=[-h0*qdot2 -h0*(qdot1+qdot2); h0*qdot1 0];

%Calculate sDelta
% sDelta_dot=-H\(C+KD)*sDelta+H\delta_tau;
sDelta_dot=-H0\(C0+KD)*sDelta+H0\delta_tau;
% sDelta_dot=-1*eye(2,2)*sDelta+1*eye(2,2)*delta_tau;
